simulink subsystem "Coral_Arm_Motor_Control_sub"  (R2023b)
settings: Solver=VariableStepAuto  StartTime=0.0  StopTime=10.0  RelTol=1e-3
undefined symbols (not defined in the file): Coral_Arm_Angle_Neg_Threshold, Coral_Arm_DC_Lower_Limit_Angle_In, Coral_Arm_DC_Lower_Limit_Out, Coral_Arm_DC_Upper_Limit_Angle_In, Coral_Arm_DC_Upper_Limit_Out, Coral_Arm_Elevator_Height_Low_Thresh, Coral_Arm_Gain_Int, Coral_Arm_Gain_Prop, Coral_Arm_Int_IC, Coral_Arm_Int_LL, Coral_Arm_Int_UL, Coral_Arm_Lower_Limit_Elevator_Height_Input, Coral_Arm_Lower_Limit_Out, Coral_Arm_Neg90_DC
libraries: simulink x6, Controls_Components_lib x1
settings Model: Creator=ander  LastModifiedBy=ander

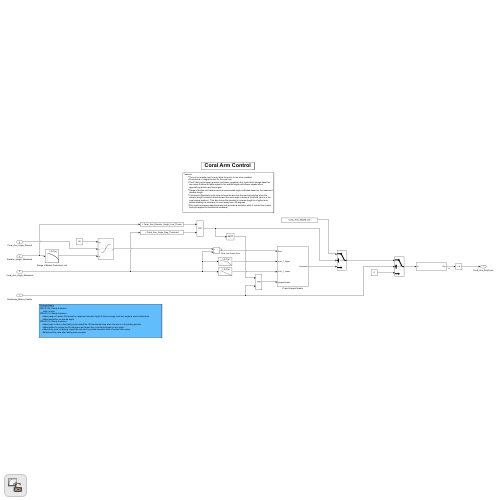
[thumbnail: Simulink's stored preview of the top-level diagram]
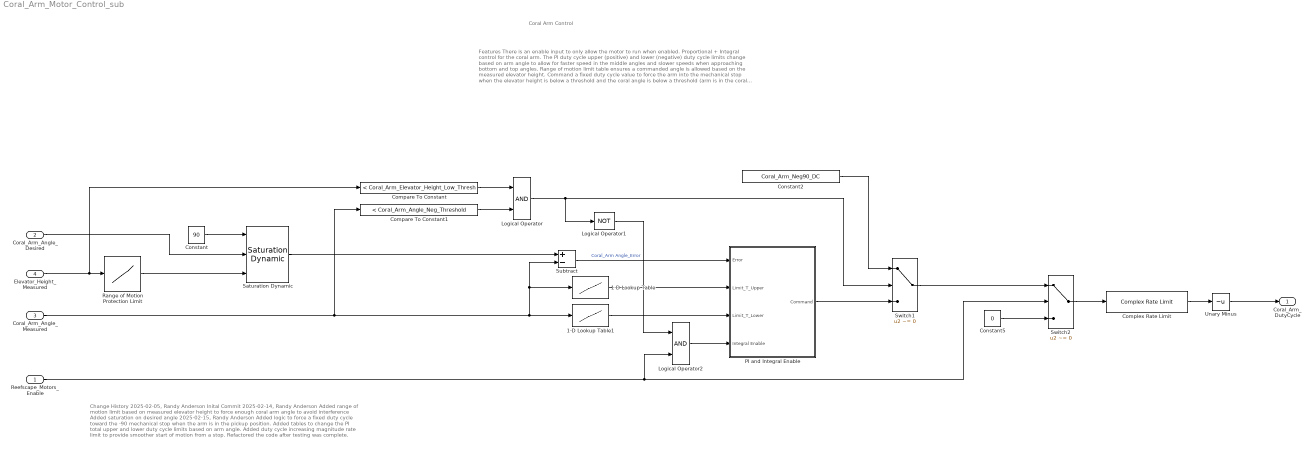
== system Coral_Arm_Motor_Control_sub ==
  note: Change History
      | 2025-02-05, Randy Anderson
      | Inital Commit
      | 2025-02-14, Randy Anderson
      | Added range of motion limit based on measured elevator height to force enough coral arm angle to avoid interference
      | Added saturation on desired angle
      | 2025-02-15, Randy Anderson
      | Added logic to force a fixed duty cycle toward the -90 mechanical stop when the arm is in the pickup position.
      | Added tables to change the PI total upper and lower duty cycle limits based on arm angle.
      | Added duty cycle increasing magnitude rate limit to provide smoother start of motion from a stop.
      | Refactored the code after testing was complete.
  note: Features
      | There is an enable input to only allow the motor to run when enabled.
      | Proportional + Integral control for the coral arm.
      | The PI duty cycle upper (positive) and lower (negative) duty cycle limits change based on arm angle to allow for faster speed in the middle angles and slower speeds when approaching bottom and top angles.
      | Range of motion limit table ensures a commanded angle is allowed based on the measured elevator height.
      | Command a fixed duty cycle value to force the arm into the mechanical stop when the elevator height is below a threshold and the coral angle is below a threshold (arm is in the coral pickup position). This also forces the elevator to increase height to a higher level before allowing the coral arm to move away from -90 degrees.
      | Duty cycle increasing magnitude rate limit provides a smoother start of motion from a stop (less jerk applied to mechanical hardware).
  note: Coral Arm Control
  Reefscape_Motors_Enable : Inport
  Coral_Arm_Angle_Desired : Inport  Port=2
  Coral_Arm_Angle_Measured : Inport  Port=3
  Elevator_Height_Measured : Inport  Port=4
  1-D Lookup Table : Lookup_n-D  NumberOfTableDimensions=1  BreakpointsForDimension1=Coral_Arm_DC_Upper_Limit_Angle_In  Table=Coral_Arm_DC_Upper_Limit_Out  ExtrapMethod=Clip  InternalRulePriority=Speed  RndMeth=Simplest
  1-D Lookup Table1 : Lookup_n-D  NumberOfTableDimensions=1  BreakpointsForDimension1=Coral_Arm_DC_Lower_Limit_Angle_In  Table=Coral_Arm_DC_Lower_Limit_Out  ExtrapMethod=Clip  InternalRulePriority=Speed  RndMeth=Simplest
  Compare To Constant : simulink/Logic and Bit Operations/Compare To Constant  relop=<  const=Coral_Arm_Elevator_Height_Low_Thresh  OutDataTypeStr=boolean
  Compare To Constant1 : simulink/Logic and Bit Operations/Compare To Constant  relop=<  const=Coral_Arm_Angle_Neg_Threshold  OutDataTypeStr=boolean
  Complex Rate Limit : Controls_Components_lib/Complex Rate Limit  Rate_Limit_Inc=Coral_Arm_DC_Inc_RL  Rate_Limit_Dec=-1  Approaching_Zero_Error_Threshold=0.01  Approaching_Zero_Final_Scale_Factor=1  Approaching_NonZero_Error_Threshold=0.01  Approaching_NonZero_Final_Scale_Factor=1
  Constant : Constant  Value=90
  Constant2 : Constant  Value=Coral_Arm_Neg90_DC
  Constant5 : Constant  Value=0
  Logical Operator : Logic  AllPortsSameDT=off  OutDataTypeStr=boolean
  Logical Operator1 : Logic  Operator=NOT  AllPortsSameDT=off  OutDataTypeStr=boolean
  Logical Operator2 : Logic  AllPortsSameDT=off  OutDataTypeStr=boolean
  PI and Integral Enable : Subsystem  mask{Gain_P=Coral_Arm_Gain_Prop, Gain_I=Coral_Arm_Gain_Int, Integral_IC=Coral_Arm_Int_IC, Limit_I_Upper=Coral_Arm_Int_UL, Limit_I_Lower=Coral_Arm_Int_LL}
      mask prompts: Gain_P "Proportional Gain"; Gain_I "Integral Gain"; Integral_IC "Integral Initial Condition"; Limit_I_Upper "Integral Upper Limit"; Limit_I_Lower "Integral Lower Limit"
  Range of Motion Protection Limit : Lookup_n-D  NumberOfTableDimensions=1  BreakpointsForDimension1=Coral_Arm_Lower_Limit_Elevator_Height_Input  Table=Coral_Arm_Lower_Limit_Out  ExtrapMethod=Clip  InternalRulePriority=Speed  RndMeth=Simplest
  Saturation Dynamic : simulink/Discontinuities/Saturation Dynamic  OutMin=[]  OutMax=[]  OutDataTypeStr=Inherit: Same as second input  OutDataType=fixdt(1, 16)  OutScaling=2^-10  DoSatur=off
  Subtract : Sum  Inputs=+-
  Switch1 : Switch  Criteria=u2 ~= 0  SaturateOnIntegerOverflow=off  InputSameDT=off
  Switch2 : Switch  Criteria=u2 ~= 0  SaturateOnIntegerOverflow=off  InputSameDT=off
  Unary Minus : UnaryMinus
  Coral_Arm_DutyCycle : Outport
  wires:
  Reefscape_Motors_Enable/1 -> Switch2/2, Logical Operator2/2
  Subtract/1 -> PI and Integral Enable/1(Error)  "Coral_Arm Angle_Error"
  Coral_Arm_Angle_Measured/1 -> Compare To Constant1/1, 1-D Lookup Table1/1, Subtract/2, 1-D Lookup Table/1
  Constant5/1 -> Switch2/3
  Switch2/1 -> Complex Rate Limit/1
  Unary Minus/1 -> Coral_Arm_DutyCycle/1
  Elevator_Height_Measured/1 -> Range of Motion Protection Limit/1, Compare To Constant/1
  Coral_Arm_Angle_Desired/1 -> Saturation Dynamic/2
  Constant/1 -> Saturation Dynamic/1
  Compare To Constant/1 -> Logical Operator/1
  Compare To Constant1/1 -> Logical Operator/2
  Range of Motion Protection Limit/1 -> Saturation Dynamic/3
  Saturation Dynamic/1 -> Subtract/1
  Switch1/1 -> Switch2/1
  PI and Integral Enable/1(Command) -> Switch1/3
  Constant2/1 -> Switch1/1
  Complex Rate Limit/1 -> Unary Minus/1
  1-D Lookup Table/1 -> PI and Integral Enable/2(Limit_T_Upper)
  1-D Lookup Table1/1 -> PI and Integral Enable/3(Limit_T_Lower)
  Logical Operator/1 -> Logical Operator1/1, Switch1/2
  Logical Operator2/1 -> PI and Integral Enable/4(Integral Enable)
  Logical Operator1/1 -> Logical Operator2/1

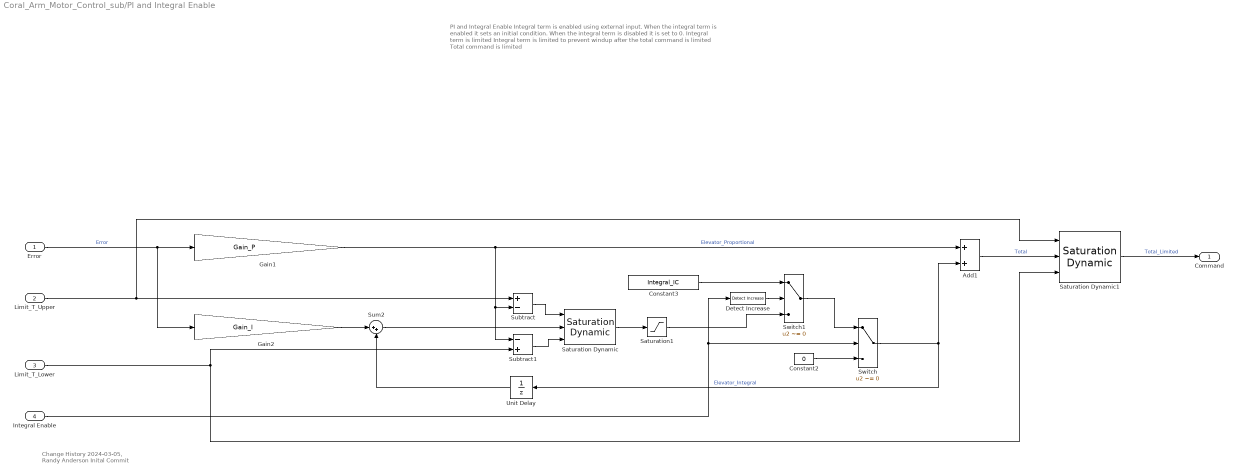
== system Coral_Arm_Motor_Control_sub/PI and Integral Enable ==
  note: Change History
      | 2024-03-05, Randy Anderson
      | Inital Commit
  note: PI and Integral Enable
      |
      | Integral term is enabled using external input.
      | When the integral term is enabled it sets an initial condition.
      | When the integral term is disabled it is set to 0.
      |
      | Integral term is limited
      |
      | Integral term is limited to prevent windup after the total command is limited
      |
      | Total command is limited
  Error : Inport
  Limit_T_Upper : Inport  Port=2
  Limit_T_Lower : Inport  Port=3
  Integral Enable : Inport  Port=4
  Add1 : Sum  Inputs=2
  Constant2 : Constant  Value=0
  Constant3 : Constant  Value=Integral_IC
  Detect Increase : simulink/Logic and Bit Operations/Detect Increase  vinit=0.0  OutDataTypeStr=boolean
  Gain1 : Gain  Gain=Gain_P
  Gain2 : Gain  Gain=Gain_I
  Saturation Dynamic : simulink/Discontinuities/Saturation Dynamic  OutMin=[]  OutMax=[]  OutDataTypeStr=Inherit: Same as second input  OutDataType=fixdt(1, 16)  OutScaling=2^-10  DoSatur=off
  Saturation Dynamic1 : simulink/Discontinuities/Saturation Dynamic  OutMin=[]  OutMax=[]  OutDataTypeStr=Inherit: Same as second input  OutDataType=fixdt(1, 16)  OutScaling=2^-10  DoSatur=off
  Saturation1 : Saturate  UpperLimit=Limit_I_Upper  LowerLimit=Limit_I_Lower
  Subtract : Sum  Inputs=+-
  Subtract1 : Sum  Inputs=-+
  Sum2 : Sum  Inputs=|++
  Switch : Switch  Criteria=u2 ~= 0  SaturateOnIntegerOverflow=off  InputSameDT=off
  Switch1 : Switch  Criteria=u2 ~= 0  SaturateOnIntegerOverflow=off  InputSameDT=off
  Unit Delay : UnitDelay  SampleTime=-1  HasFrameUpgradeWarning=on
  Command : Outport
  wires:
  Constant3/1 -> Switch1/1
  Saturation1/1 -> Switch1/3
  Detect Increase/1 -> Switch1/2
  Switch1/1 -> Switch/1
  Switch/1 -> Add1/2, Unit Delay/1  "Elevator_Integral"
  Saturation Dynamic1/1 -> Command/1  "Total_Limited"
  Sum2/1 -> Saturation Dynamic/2
  Add1/1 -> Saturation Dynamic1/2  "Total"
  Limit_T_Lower/1 -> Subtract1/2, Saturation Dynamic1/3
  Limit_T_Upper/1 -> Subtract/1, Saturation Dynamic1/1
  Unit Delay/1 -> Sum2/2
  Subtract/1 -> Saturation Dynamic/1
  Saturation Dynamic/1 -> Saturation1/1
  Gain2/1 -> Sum2/1
  Gain1/1 -> Subtract/2, Subtract1/1, Add1/1  "Elevator_Proportional"
  Subtract1/1 -> Saturation Dynamic/3
  Error/1 -> Gain1/1, Gain2/1  "Error"
  Integral Enable/1 -> Switch/2, Detect Increase/1
  Constant2/1 -> Switch/3
